simulink model "HIL"  (R2024a)
settings: Solver=FixedStepAuto  StartTime=0.0  StopTime=inf  FixedStep=0.005  RelTol=1e-3  EnableMultiTasking=on
values from neighbouring files (symbols this model uses):
  K_lqr = lqr(A,B,Q,R)    [lqr_script.m]
libraries: arduinolib x2, simulink_extras x2, arduinosensorlib x2, eeGeneralControl x2
settings Model: FPTRunName=Active  ExtModeTrigDuration=2  Creator=Mostafa  LastModifiedBy=Mostafa
settings SolverCC: AlgebraicLoopSolver=TrustRegion  AutoInsertRateTranBlk=on
settings DataIOCC: LimitDataPoints=on  SaveFormat=Array
settings OptimizationCC: ReuseModelBlockBuffer=off  ExpressionDepthLimit=2147483647  LifeSpan=Inf  MaxStackSize=64
settings DebuggingCC: UnderspecifiedInitializationDetection=Classic  MergeDetectMultiDrivingBlocksExec=none  FcnCallInpInsideContextMsg=warning  UnconnectedInputMsg=warning  UnconnectedOutputMsg=warning  UnconnectedLineMsg=warning  AllowSymbolicDim=off  StateNameClashWarn=warning  SFUnexpectedBacktrackingDiag=warning  SFNoUnconditionalDefaultTransitionDiag=warning  SFExecutionAtInitializationDiag=none  ArithmeticOperatorsInVariantConditions=warning
settings HardwareCC: ProdBitPerPointer=32  ProdBitPerSizeT=32  ProdBitPerPtrDiffT=32  ProdLargestAtomicInteger=Long  ProdLargestAtomicFloat=Double  ProdWordSize=32  ProdHWDeviceType=ARM Compatible->ARM Cortex
settings ModelReferenceCC: EnableRefExpFcnMdlSchedulingChecks=on  PropagateSignalLabelsOutOfModel=off
settings SFSimCC: SimUseLocalCustomCode=off  CustomCodeUndefinedFunction=UseInterfaceOnly
settings RTWCC: Description=Embedded Coder  SystemTargetFile=ert.tlc  HardwareBoard=ESP32-WROOM(Arduino Compatible)  TemplateMakefile=ert_default_tmf  RTWVerbose=off  RTWUseLocalCustomCode=off  Toolchain=ESP32  BuildConfiguration=Faster Runs  GPUComputeCapability=3.5
settings CodeAppCC: ForceParamTrailComments=on  OperatorAnnotations=on  StateflowObjectComments=on  MATLABSourceComments=on
settings ERTTargetCC: MultiwordLength=2048  ERTCustomFileBanners=off  SupportContinuousTime=on  SupportNonInlinedSFcns=on  RemoveResetFunc=off  SupportVariableSizeSignals=on  ModelStepFunctionPrototypeControlCompliant=off  ExtModeTransport=3  ExtModeStaticAlloc=on  ExtModeAutomaticAllocSize=off  ExtModeStaticAllocSize=65536  ExtModeMexFile=ext_xcp  ExtModeIntrfLevel=Level2 - Open
settings ConfigComp: CovMetricSettings=dw  CovSaveCumulativeToWorkspaceVar=on  CovSaveSingleToWorkspaceVar=on  CovExternalEMLEnable=off  CovSFcnEnable=off

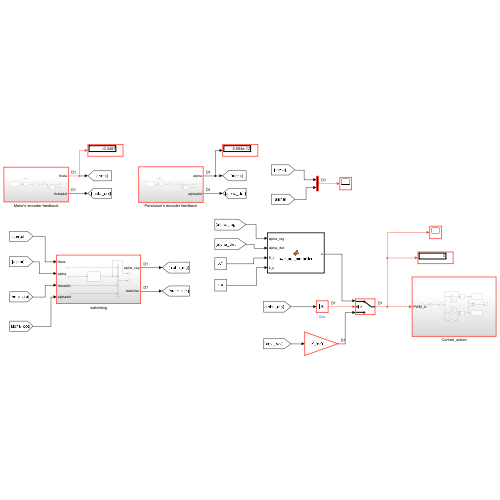
[thumbnail: Simulink's stored preview of the top-level diagram]
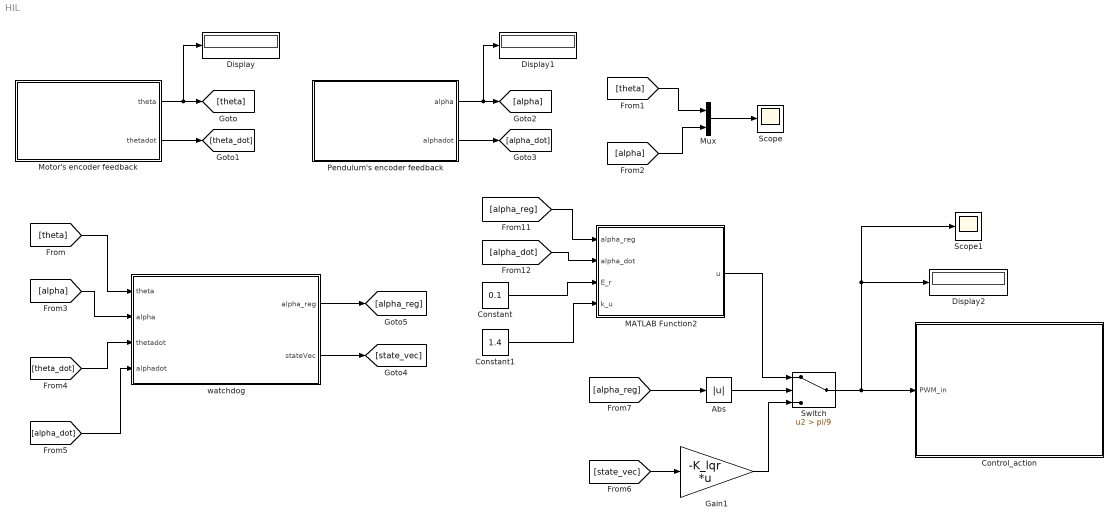
== system HIL ==
  Abs : Abs  SaturateOnIntegerOverflow=off
  Constant : Constant  Value=0.1
  Constant1 : Constant  Value=1.4
  Control_action : Subsystem
  Display : Display
  Display1 : Display
  Display2 : Display
  Gain1 : Gain  Gain=-K_lqr  Multiplication=Matrix(K*u)
  MATLAB Function2 : MATLAB Function  TreatAsAtomicUnit=on
  Motor's encoder feedback : Subsystem
  Mux : Mux  Inputs=2
  Pendulum's encoder feedback : Subsystem
  Scope : Scope
  Scope1 : Scope
  Switch : Switch  Criteria=u2 > Threshold  Threshold=pi/9  SaturateOnIntegerOverflow=off  InputSameDT=off
  watchdog : Subsystem
  wires:
  Switch/1 -> Scope1/1, Display2/1, Control_action/1(PWM_in)
  MATLAB Function2/1(u) -> Switch/1
  Abs/1 -> Switch/2
  Gain1/1 -> Switch/3
  Mux/1 -> Scope/1
  Motor's encoder feedback/1(theta) -> Display/1, [theta]
  [theta] -> watchdog/1(theta)
  Motor's encoder feedback/2(thetadot) -> [theta_dot]
  Pendulum's encoder feedback/2(alphadot) -> [alpha_dot]
  Pendulum's encoder feedback/1(alpha) -> Display1/1, [alpha]
  [theta] -> Mux/1
  [alpha] -> Mux/2
  [alpha] -> watchdog/2(alpha)
  [theta_dot] -> watchdog/3(thetadot)
  [alpha_dot] -> watchdog/4(alphadot)
  Constant1/1 -> MATLAB Function2/4(k_u)
  Constant/1 -> MATLAB Function2/3(E_r)
  [alpha_reg] -> MATLAB Function2/1(alpha_reg)
  [alpha_dot] -> MATLAB Function2/2(alpha_dot)
  watchdog/2(stateVec) -> [state_vec]
  watchdog/1(alpha_reg) -> [alpha_reg]
  [state_vec] -> Gain1/1
  [alpha_reg] -> Abs/1

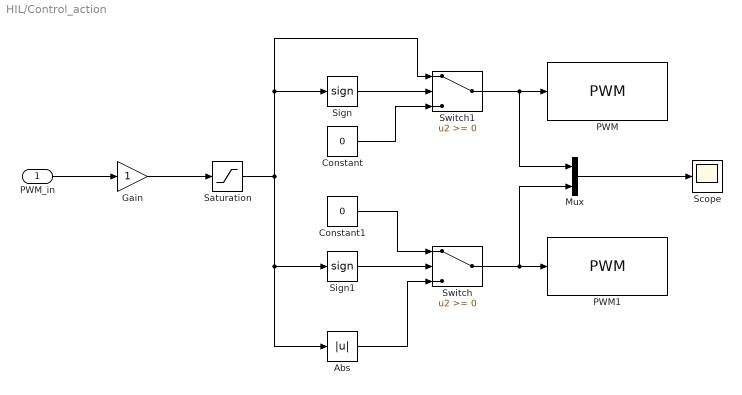
== system HIL/Control_action ==
  PWM_in : Inport
  Abs : Abs  SaturateOnIntegerOverflow=off
  Constant : Constant  Value=0
  Constant1 : Constant  Value=0
  Gain : Gain
  Mux : Mux  Inputs=2
  PWM : arduinolib/PWM  pinNumber=18  frequencyType=Default  desiredFrequency=490.2  achievableFrequency=490.2
  PWM1 : arduinolib/PWM  pinNumber=19  frequencyType=Default  desiredFrequency=490.2  achievableFrequency=490.2
  Saturation : Saturate  UpperLimit=255  LowerLimit=-255
  Scope : Scope
  Sign : Signum
  Sign1 : Signum
  Switch : Switch  SaturateOnIntegerOverflow=off  InputSameDT=off
  Switch1 : Switch  SaturateOnIntegerOverflow=off  InputSameDT=off
  wires:
  Constant1/1 -> Switch/1
  Abs/1 -> Switch/3
  Gain/1 -> Saturation/1
  Mux/1 -> Scope/1
  Switch1/1 -> Mux/1, PWM/1
  Switch/1 -> Mux/2, PWM1/1
  PWM_in/1 -> Gain/1
  Constant/1 -> Switch1/3
  Saturation/1 -> Sign1/1, Abs/1, Sign/1, Switch1/1
  Sign/1 -> Switch1/2
  Sign1/1 -> Switch/2

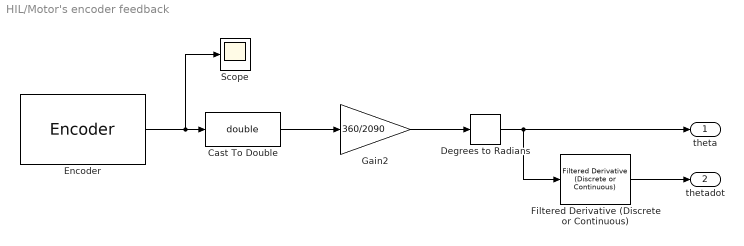
== system HIL/Motor's encoder feedback ==
  Cast To Double : DataTypeConversion  OutDataTypeStr=double  SaturateOnIntegerOverflow=off  RndMeth=Floor
  Degrees to Radians : simulink_extras/Transformations/Degrees to Radians
  Encoder : arduinosensorlib/Encoder  InputA=22  InputB=23  Mode=No reset  SampleTime=0.005
  Filtered Derivative (Discrete or Continuous) : eeGeneralControl/Filtered Derivative (Discrete or Continuous)  K=1  T=0.03  B=inf  A=-inf  minRatio=10  init_option=Inherited from block input  x0=0  Ts=-1
      settings: LibrarySourceBlock=|
      | ee_sl_lib/General Control/Filtered Derivative
      | (Discrete or Continuous)
  Gain2 : Gain  Gain=360/2090
  Scope : Scope
  theta : Outport
  thetadot : Outport  Port=2
  wires:
  Encoder/1 -> Scope/1, Cast To Double/1
  Cast To Double/1 -> Gain2/1
  Degrees to Radians/1 -> Filtered Derivative (Discrete or Continuous)/1, theta/1
  Gain2/1 -> Degrees to Radians/1
  Filtered Derivative (Discrete or Continuous)/1 -> thetadot/1

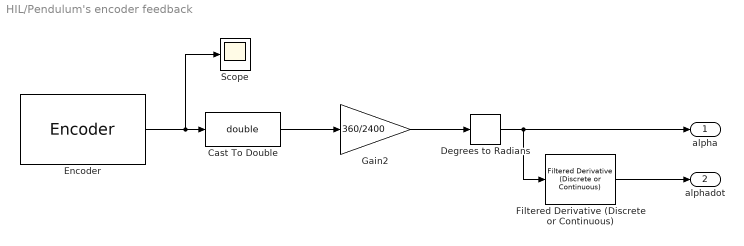
== system HIL/Pendulum's encoder feedback ==
  Cast To Double : DataTypeConversion  OutDataTypeStr=double  SaturateOnIntegerOverflow=off  RndMeth=Floor
  Degrees to Radians : simulink_extras/Transformations/Degrees to Radians
  Encoder : arduinosensorlib/Encoder  InputA=32  InputB=33  Mode=No reset  SampleTime=0.005
  Filtered Derivative (Discrete or Continuous) : eeGeneralControl/Filtered Derivative (Discrete or Continuous)  K=1  T=0.03  B=inf  A=-inf  minRatio=10  init_option=Inherited from block input  x0=0  Ts=-1
      settings: LibrarySourceBlock=|
      | ee_sl_lib/General Control/Filtered Derivative
      | (Discrete or Continuous)
  Gain2 : Gain  Gain=360/2400
  Scope : Scope
  alpha : Outport
  alphadot : Outport  Port=2
  wires:
  Encoder/1 -> Scope/1, Cast To Double/1
  Cast To Double/1 -> Gain2/1
  Degrees to Radians/1 -> Filtered Derivative (Discrete or Continuous)/1, alpha/1
  Gain2/1 -> Degrees to Radians/1
  Filtered Derivative (Discrete or Continuous)/1 -> alphadot/1

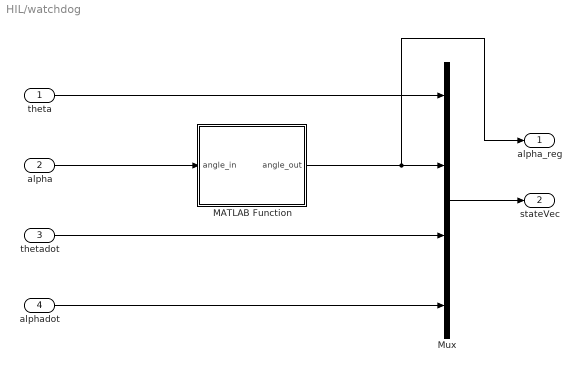
== system HIL/watchdog ==
  theta : Inport
  alpha : Inport  Port=2
  thetadot : Inport  Port=3
  alphadot : Inport  Port=4
  MATLAB Function : MATLAB Function  TreatAsAtomicUnit=on
  Mux : Mux
  alpha_reg : Outport
  stateVec : Outport  Port=2
  wires:
  thetadot/1 -> Mux/3
  theta/1 -> Mux/1
  alpha/1 -> MATLAB Function/1(angle_in)
  MATLAB Function/1(angle_out) -> alpha_reg/1, Mux/2
  Mux/1 -> stateVec/1
  alphadot/1 -> Mux/4

== matlab function HIL/MATLAB Function2 ==
  data: alpha_reg input; u output; alpha_dot input; E_r input; k_u input
function u = swingup_controller(alpha_reg, alpha_dot,E_r,k_u)

    M_p = 0.0075;   % Mass of pendulum (kg)
    L_p = 0.1;      % Length to COM (m)
    J_p = 0.0015;   % Inertia (kg*m^2)
    g   = 9.81;
  
    E_total = M_p * g * L_p * (1 - cos(alpha_reg)) + 0.5 * J_p * alpha_dot^2;    
    u_swing = k_u * (E_r - E_total) * alpha_dot * cos(alpha_reg);
    
    % Saturation limits
    if u_swing > 200; u_swing = 200; end
    if u_swing < -200; u_swing = -200; end

    u = u_swing;
end

== matlab function HIL/watchdog/MATLAB Function ==
  data: angle_in input; angle_out output
function angle_out = wrap_angle(angle_in)
    % This wraps any angle (in radians) to the range [-pi, pi]
    angle_out = atan2(sin(angle_in - pi), cos(angle_in - pi));
end
